simulink model "PILEncoder"  (R2021a)
settings: Solver=FixedStepAuto  StartTime=0.0  StopTime=41.24  FixedStep=0.001  RelTol=1e-3  EnableMultiTasking=on
values from neighbouring files (symbols this model uses):
  den_lpf_d = den_lpf20    [Mainframe_init.m]    (also in load_autopilot.m)
  Emulated_FCC_IO_Delay = 7    [Mainframe_init.m]
  Enable_Gyros = 0    [Mainframe_init.m]
  Enable_INS = 0    [Mainframe_init.m]
  num_lpf_d = num_lpf20    [Mainframe_init.m]    (also in load_autopilot.m)
undefined symbols (not defined in the file or in its folder): act_dmp, act_omega, Actuator, Aerodynamics, aMode, Autopilot, AUX, c_b_WGS, c_be, c_flat, c_grav, c_h_geop0, c_h_geope, c_pa0, c_pe, c_r0, c_rot, c_rsma, c_Tmp0, d_siB_0, d_siB_max, d_siB_min, dd_siB_max, dd_siB_min, dev, DiscIntNeverNeededParam, e_pa, e_Tmp, Earth, fin_maxrate, flag_I_act_switch, flag_I_aero_switch, flag_I_flat, flag_I_gravity_switch, flag_I_rot, Flight_Logic, hcr, HIL_Data, JMMM_0, JMMM_e, JSPB_e, lat_0, lon_0, Main, Mass_Props, mB_0, mM_0, mM_e, pBII_0, pMPB, pNPB, propellant_kg, prp_FBPB, prp_mdot, prp_T, pSPB, pwm_output0, pwm_output1, qEG_0, qIB_0 ... (+30)
libraries: simulink x42, simulink_extras x24, aerolibcommonsys x4, px4lib x2, custom_blocks x1, dspstat3 x1, pil_lib x1, aerolibtransform2 x1, dspnetwork x1, aerolibnav x1
(part 6 of 16)

== system PILEncoder/Non-linear Flight Dynamic Model/Subsystem1/GRM_Airframe/gravity/launch_rail ==
  gBG_c : Inport
  hBE : Inport  Port=2
  Constant1 : Constant  Value=flag_I_gravity_switch
  Constant3 : Constant  Value=0
  Subtract : Sum  Inputs=++-
  Switch : Switch  Criteria=u2 > Threshold  Threshold=0.05
  Vector Concatenate : Concatenate  NumInputs=3
  initial_altitude : Subsystem
  gBG : Outport  VectorParamsAs1DForOutWhenUnconnected=off
  wires:
  Constant1/1 -> Subtract/2
  hBE/1 -> Subtract/1
  Subtract/1 -> Switch/2
  Constant3/1 -> Vector Concatenate/1, Vector Concatenate/2, Vector Concatenate/3
  Switch/1 -> gBG/1  "gBG"
  Vector Concatenate/1 -> Switch/3
  gBG_c/1 -> Switch/1
  initial_altitude/1(hBE_0) -> Subtract/3

== system PILEncoder/Non-linear Flight Dynamic Model/Subsystem1/GRM_Airframe/motion_kinematics/calc_motion_kinematics ==
  lat : Inport
  lon : Inport  Port=2
  qIB : Inport  Port=3
  calc_transformation_matrix : Subsystem
  earth_rotation : Subsystem
  wIEE : Outport  VectorParamsAs1DForOutWhenUnconnected=off
  TIE : Outport  Port=2  VectorParamsAs1DForOutWhenUnconnected=off
  TEB : Outport  Port=3  VectorParamsAs1DForOutWhenUnconnected=off
  TGB : Outport  Port=4  VectorParamsAs1DForOutWhenUnconnected=off
  TEG : Outport  Port=5  VectorParamsAs1DForOutWhenUnconnected=off
  wEGG : Outport  Port=6  VectorParamsAs1DForOutWhenUnconnected=off
  TIB : Outport  Port=7  VectorParamsAs1DForOutWhenUnconnected=off
  wires:
  earth_rotation/1(wIEE) -> wIEE/1
  earth_rotation/2(TIE) -> TIE/1
  earth_rotation/5(TEG) -> TEG/1
  earth_rotation/6(wEGG) -> wEGG/1
  lon/1 -> earth_rotation/2(lon)
  lat/1 -> earth_rotation/1(lat)
  earth_rotation/3(qIE) -> calc_transformation_matrix/1(qIE)
  earth_rotation/4(qEG) -> calc_transformation_matrix/2(qEG)
  qIB/1 -> calc_transformation_matrix/3(qIB)
  calc_transformation_matrix/1(TEB) -> TEB/1
  calc_transformation_matrix/2(TGB) -> TGB/1
  calc_transformation_matrix/3(TIB) -> TIB/1

== system PILEncoder/Non-linear Flight Dynamic Model/Subsystem1/GRM_Airframe/propulsion/prp_look_up ==
  env_glbl_bus : Inport
  Bus Selector1 : BusSelector  OutputSignals=T_sim_glbl,T_sim_lnch
  Constant : Constant  Value=0
  Constant1 : Constant  Value=0
  Saturation : Saturate  UpperLimit=prp_T(end)  LowerLimit=0
      settings: AttributesFormatString=|
      | %<UpperLimit>
      | %<LowerLimit>
  Subtract : Sum  Inputs=+-
  Switch : Switch  Criteria=u2 > Threshold
  Switch1 : Switch  Criteria=u2 > Threshold
  Vector Concatenate : Concatenate  NumInputs=3
  thrust_lookup : Lookup_n-D  NumberOfTableDimensions=1  BreakpointsForDimension1=prp_T  Table=prp_FBPB  ExtrapMethod=Clip  UseLastTableValue=on  InternalRulePriority=Speed  RndMeth=Simplest  InputSameDT=on
  FBPM : Outport  VectorParamsAs1DForOutWhenUnconnected=off
  wires:
  Bus Selector1/2 -> Subtract/2  "<T_sim_lnch>"
  Switch/1 -> Saturation/1, Switch1/2, Switch1/3
  thrust_lookup/1 -> Switch1/1
  Bus Selector1/1 -> Subtract/1  "<T_sim_glbl>"
  env_glbl_bus/1 -> Bus Selector1/1
  Constant/1 -> Switch/3
  Subtract/1 -> Switch/1, Switch/2
  Saturation/1 -> thrust_lookup/1
  Vector Concatenate/1 -> FBPM/1  "FBPM"
  Constant1/1 -> Vector Concatenate/3, Vector Concatenate/2
  Switch1/1 -> Vector Concatenate/1  "a_FBPM"

== system PILEncoder/Non-linear Flight Dynamic Model/Subsystem1/GRM_Airframe/propulsion/prp_uncertainty ==
  FBPM : Inport
  wab : Inport  Port=2
  3_rot_mat : Subsystem  mask(Rotation um 1, 2 oder 3 Achsen){rot_1=Rotation um z-Achse, rot_2=Rotation um y-Achse, rot_3=Rotation um x-Achse}
      mask prompts: rot_1 "1. Rotation"; rot_2 "2. Rotation"; rot_3 "3. Rotation"
      mask help:
      | Dieser Block liefert die Rotationsmatrix T12 für den Fall zurück, dass sich das Ziel-Koordinatensystem (1) durch Drehungen um 1, 2 oder 3 Achsen gegenüber dem Ausgangskoordinatensystem (2) beschreiben lässt (passive Drehung).
      |
      | Die Anzahl der Rotation sowie die Reihenfolge ist frei einstellbar.
      |
      | Die Rotationswinkel haben die Einheit [rad].
      mask TypeOptions rot_1: Rotation um x-Achse | Rotation um y-Achse | Rotation um z-Achse
      mask TypeOptions rot_2: Rotation um x-Achse | Rotation um y-Achse | Rotation um z-Achse
      mask TypeOptions rot_3: Rotation um x-Achse | Rotation um y-Achse | Rotation um z-Achse
  Bus Selector : BusSelector  OutputSignals=pBPB
  Product : Product  Multiplication=Matrix(*)
  Product1 : Product
  Subtract : Sum  Inputs=+-
  Thrust_rot_z : Constant  Value=unc_prp_z
  cross_product : Subsystem
      mask help: cross product r3 = r1 x r2
      mask Help:
      | Name:
      | 
      |     cross_product
      | 
      | Description:
      | 
      |     This block implements the cross product r3 = r1 x r2.
      | 
      | Inputs  [size] [data type] [unit]:
      | 
      |     vector 1  [3] [double] [-]
      |     vector 2  [3] [double] [-]
      | 
      | Outputs  [size] [data type] [unit]:
      | 
      |     resulting vector  [3] [double] [-]
      mask Display: disp(' r3 = r1 x r2')
  pNPB : Constant  Value=pNPB
  thrust_rot_x : Constant  Value=unc_prp_x
  thrust_rot_y : Constant  Value=unc_prp_y
  uncert_thrust : Constant  Value=unc_prp_scale
  FBPB : Outport  VectorParamsAs1DForOutWhenUnconnected=off
  MBPB : Outport  Port=2  VectorParamsAs1DForOutWhenUnconnected=off
  wires:
  Thrust_rot_z/1 -> 3_rot_mat/1(wi1)
  thrust_rot_x/1 -> 3_rot_mat/3(wi3)
  Product/1 -> cross_product/2(r2), FBPB/1  "FBPB"
  FBPM/1 -> Product1/1
  3_rot_mat/1(T12) -> Product/1
  thrust_rot_y/1 -> 3_rot_mat/2(wi2)
  cross_product/1(r1_x_r2) -> MBPB/1  "MBPB"
  wab/1 -> Bus Selector/1
  Bus Selector/1 -> Subtract/1  "<pBPB>"
  uncert_thrust/1 -> Product1/2
  Product1/1 -> Product/2
  pNPB/1 -> Subtract/2
  Subtract/1 -> cross_product/1(r1)

== system PILEncoder/Non-linear Flight Dynamic Model/Subsystem1/GRM_Airframe/rb_eom/calc_bus_flight_dyn_bus_entries ==
  mot_kin : Inport
  eom : Inport  Port=2
  Bus Selector : BusSelector  OutputSignals=pBII,vBII,qIB,wBIB,d_wBIB,d_vBII
  Bus Selector1 : BusSelector  OutputSignals=pBII
  Bus Selector3 : BusSelector  OutputSignals=TGB,TIB,TIE
  Constant : Constant  Value=pBII_0
      settings: AttributesFormatString=%<Value>
  Gain : Gain  Gain=-1
  Math Function : Math  Operator=transpose  SignedPower=on  SaturateOnIntegerOverflow=on
  Product{,1..3} (4 alike) : Product  Multiplication=Matrix(*)
  Subsystem2 : Subsystem
  Sum : Sum  Inputs=+-
  eom D1 : InportShadow  Port=2
  q12_from_T12 : Subsystem
      mask help: Transforms a Direction Cosine Matrix into a Quaternion
      mask Help:
      | Name:
      | 
      |     q12_from_T12
      | 
      | Description:
      | 
      |     This block implements the transformation of a direction cosine matrix DCM
      |      into the corresponding quaternion.
      | 
      | Inputs  [size] [data type] [unit]:
      | 
      |     direction cosine matrix T12  [3x3] [double] [-]
      | 
      | Outputs  [size] [data type] [unit]:
      | 
      |     quaternion q12  [4] [double] [-]
      mask Display:
      | %port_label('input', 1, 'T12')
      | %port_label('output', 1, 'q12')
      | disp('DCM \rightarrow q','texmode','on')
  quaternion_to_euler_angles : Subsystem
      mask help: transforms quaternions to Euler angles (roll, pitch, yaw)
      mask Help:
      | Name:
      | 
      |     quaternion_to_euler_angles
      | 
      | Description:
      | 
      |     This block implements the transformation of a quaternion into the
      |     corresponding Euler angles (zyx-sequence, roll, pitch, yaw).
      | 
      | Inputs  [size] [data type] [unit]:
      | 
      |     quaternion  [4] [double] [-]
      | 
      | Outputs  [size] [data type] [unit]:
      | 
      |     roll angle phi  [1] [double] [rad]
      |     pitch angle theta  [1] [double] [rad]
      |     yaw angle psi  [1] [double] [rad]
      mask Display:
      | %disp (' q --> (Phi,Theta,Psi) [rad]')
      | disp('q \rightarrow eu(\Phi;\Theta;\Psi)','texmode','on')
  quaternion_to_euler_angles1 : Subsystem
      mask help: transforms quaternions to Euler angles (roll, pitch, yaw)
      mask Help:
      | Name:
      | 
      |     quaternion_to_euler_angles
      | 
      | Description:
      | 
      |     This block implements the transformation of a quaternion into the
      |     corresponding Euler angles (zyx-sequence, roll, pitch, yaw).
      | 
      | Inputs  [size] [data type] [unit]:
      | 
      |     quaternion  [4] [double] [-]
      | 
      | Outputs  [size] [data type] [unit]:
      | 
      |     roll angle phi  [1] [double] [rad]
      |     pitch angle theta  [1] [double] [rad]
      |     yaw angle psi  [1] [double] [rad]
      mask Display:
      | %disp (' q --> (Phi,Theta,Psi) [rad]')
      | disp('q \rightarrow eu(\Phi;\Theta;\Psi)','texmode','on')
  aBIB : Outport  VectorParamsAs1DForOutWhenUnconnected=off
  lon : Outport  Port=2  VectorParamsAs1DForOutWhenUnconnected=off
  lat : Outport  Port=3  VectorParamsAs1DForOutWhenUnconnected=off
  hBE : Outport  Port=4  VectorParamsAs1DForOutWhenUnconnected=off
  vBII : Outport  Port=5  VectorParamsAs1DForOutWhenUnconnected=off
  qIB : Outport  Port=6  VectorParamsAs1DForOutWhenUnconnected=off
  wBIB : Outport  Port=7  VectorParamsAs1DForOutWhenUnconnected=off
  d_wBIB : Outport  Port=8  VectorParamsAs1DForOutWhenUnconnected=off
  d_vBII : Outport  Port=9  VectorParamsAs1DForOutWhenUnconnected=off
  pBII : Outport  Port=10  VectorParamsAs1DForOutWhenUnconnected=off
  euIB : Outport  Port=11  VectorParamsAs1DForOutWhenUnconnected=off
  vBIB : Outport  Port=12  VectorParamsAs1DForOutWhenUnconnected=off
  qGB : Outport  Port=13  VectorParamsAs1DForOutWhenUnconnected=off
  euGB : Outport  Port=14  VectorParamsAs1DForOutWhenUnconnected=off
  euBG : Outport  Port=15  VectorParamsAs1DForOutWhenUnconnected=off
  pBLG : Outport  Port=16  VectorParamsAs1DForOutWhenUnconnected=off
  wires:
  Bus Selector/1 -> pBII/1, Subsystem2/2(pBII)  "<pBII>"
  mot_kin/1 -> Bus Selector3/1
  Bus Selector3/3 -> Subsystem2/1(TIE)  "<TIE>"
  eom/1 -> Bus Selector/1
  Math Function/1 -> [TBI], Product1/1, Product/1  "TBI"
  Bus Selector3/2 -> Math Function/1  "<TIB>"
  Bus Selector/6 -> Product/2, d_vBII/1  "<d_vBII>"
  Product/1 -> aBIB/1  "aBIB"
  Subsystem2/1(lon) -> lon/1
  Subsystem2/2(lat) -> lat/1
  Subsystem2/3(hBE) -> hBE/1  "hBE"
  Bus Selector/2 -> Product1/2, vBII/1  "<vBII>"
  Bus Selector/3 -> quaternion_to_euler_angles/1(q), qIB/1  "<qIB>"
  Bus Selector/4 -> wBIB/1  "<wBIB>"
  Bus Selector/5 -> d_wBIB/1  "<d_wBIB>"
  quaternion_to_euler_angles/1(eulx) -> euIB/1  "euIB"
  Product1/1 -> vBIB/1  "vBIB"
  Bus Selector3/1 -> [TGB], q12_from_T12/1(T12)  "<TGB>"
  q12_from_T12/1(q12) -> quaternion_to_euler_angles1/1(q), qGB/1  "qGB"
  quaternion_to_euler_angles1/1(eulx) -> euGB/1, Gain/1  "euGB"
  Gain/1 -> euBG/1  "euBG"
  eom D1/1 -> Bus Selector1/1
  Bus Selector1/1 -> Sum/1  "<pBII>"
  Constant/1 -> Sum/2
  Sum/1 -> Product3/2  "pBLI"
  [TGB] -> Product2/1
  [TBI] -> Product2/2
  Product2/1 -> Product3/1  "TGI"
  Product3/1 -> pBLG/1  "pBLG"

== system PILEncoder/Non-linear Flight Dynamic Model/Subsystem1/GRM_Airframe/rb_eom/eom_6dof ==
  for_mom : Inport
  wab : Inport  Port=2
  Bus Selector1 : BusSelector  OutputSignals=mB,JBBB
  Bus Selector2 : BusSelector  OutputSignals=FBTB,MBTB
  Constant : Constant  Value=[pBII_0; vBII_0; qIB_0; wBIB_0]
  Constant9 : Constant  Value=[0 0 0; 0 0 0; 0 0 0]
  Rigid_Body_EOM_6_DOF : Subsystem  mask{flag_Kraft=FBTB}
      mask prompts: flag_Kraft "Input Kraftvektor"
      mask help:
      | 6DOF-Bewegungsgleichungen im ECI-System mit
      | zeitvariantem Massenträgheitsmoment.
      |
      | Modell Varianten:
      | - Koordinatensystem des Kraftvektor:
      |      FBTI : Inertial System I
      |      FBTB : Körperfestes System B
      mask init:
      | switch flag_Kraft
      |     case 1
      |         port_label_kraft = 'FBTI';
      |     case 2
      |         port_label_kraft = 'FBTB';
      | end
      mask TypeOptions flag_Kraft: FBTI | FBTB
      mask DialogControl Container4 Prompt: Modell Einstellungen
      mask Display:
      | port_label ('input',1,port_label_kraft )
      | port_label ('input',2,'MBTB' )
      | port_label ('input',3,'mB' )
      | port_label ('input',4,'x0' )
      | port_label ('input',5,'JBB' )
      | port_label ('input',6,'d_JBB' )
      | port_label ('output',1,'rb_eom' )
  eom : Outport  VectorParamsAs1DForOutWhenUnconnected=off
  wires:
  Bus Selector2/2 -> Rigid_Body_EOM_6_DOF/2(MBTB)  "<MBTB>"
  Bus Selector2/1 -> Rigid_Body_EOM_6_DOF/1(FBTX)  "<FBTB>"
  Rigid_Body_EOM_6_DOF/1(rb_eom) -> eom/1
  Constant9/1 -> Rigid_Body_EOM_6_DOF/6(d_JBB)
  Bus Selector1/2 -> Rigid_Body_EOM_6_DOF/5(JBB)  "<JBBB>"
  for_mom/1 -> Bus Selector2/1
  Constant/1 -> Rigid_Body_EOM_6_DOF/4(x0)
  Bus Selector1/1 -> Rigid_Body_EOM_6_DOF/3(mB)  "<mB>"
  wab/1 -> Bus Selector1/1

== system PILEncoder/Non-linear Flight Dynamic Model/Subsystem1/GRM_Airframe/stream_flow/calc_stream_flow ==
  TIB : Inport
  wIEE : Inport  Port=2
  TIE : Inport  Port=3
  VBII : Inport  Port=4
  pBII : Inport  Port=5
  wBIB : Inport  Port=6
  rho : Inport  Port=7
  sos : Inport  Port=8
  hBE : Inport  Port=9
  Bus Creator : BusCreator  Inputs=9
  Math Function : Math  Operator=transpose  SignedPower=on  SaturateOnIntegerOverflow=on
  Product : Product  Multiplication=Matrix(*)
  Subsystem1 : Subsystem
  velocity_vector_transformation : Subsystem
  str_flow : Outport  VectorParamsAs1DForOutWhenUnconnected=off
  wires:
  Subsystem1/4(MaB) -> Bus Creator/4
  Math Function/1 -> Product/1  "TBI"
  Subsystem1/2(be) -> Bus Creator/2  "beB"
  Subsystem1/8(fi) -> Bus Creator/8  "fiB"
  VBII/1 -> velocity_vector_transformation/3(vBII)
  Subsystem1/5(a_vB) -> Bus Creator/5
  Product/1 -> Subsystem1/1(vBEB)  "vBEB"
  Subsystem1/6(wBIB_star) -> Bus Creator/6
  TIE/1 -> velocity_vector_transformation/2(TIE)
  Subsystem1/3(qdynB) -> Bus Creator/3
  velocity_vector_transformation/1(vBEI) -> Product/2
  Subsystem1/7(th) -> Bus Creator/7  "inB"
  Subsystem1/1(al) -> Bus Creator/1  "alB"
  wIEE/1 -> velocity_vector_transformation/1(wIEE)
  Bus Creator/1 -> str_flow/1  "str_flow_bus"
  wBIB/1 -> Subsystem1/2(wBIB)
  hBE/1 -> Bus Creator/9
  sos/1 -> Subsystem1/4(sos)
  rho/1 -> Subsystem1/3(rho)
  TIB/1 -> Math Function/1
  pBII/1 -> velocity_vector_transformation/4(pBII)

== system PILEncoder/Non-linear Flight Dynamic Model/Subsystem1/GRM_Airframe/weight_and_balance/center_of_gravity ==
  mB : Inport
  mM : Inport  Port=2
  1-D Lookup Table : Lookup_n-D  NumberOfTableDimensions=1  BreakpointsForDimension1=Mass_Props.propellant_bkpts  Table=Mass_Props.CGx_m_tbl  ExtrapMethod=Clip  UseLastTableValue=on  InternalRulePriority=Speed  RndMeth=Simplest  InputSameDT=on
      settings: AttributesFormatString=|
      | %<Table>
      | %<BreakpointsForDimension1>
  1-D Lookup Table3 : Lookup_n-D  NumberOfTableDimensions=1  BreakpointsForDimension1=Mass_Props.propellant_bkpts  Table=Mass_Props.CGy_m_tbl  ExtrapMethod=Clip  UseLastTableValue=on  InternalRulePriority=Speed  RndMeth=Simplest  InputSameDT=on
      settings: AttributesFormatString=|
      | %<Table>
      | %<BreakpointsForDimension1>
  1-D Lookup Table6 : Lookup_n-D  NumberOfTableDimensions=1  BreakpointsForDimension1=Mass_Props.propellant_bkpts  Table=Mass_Props.CGz_m_tbl  ExtrapMethod=Clip  UseLastTableValue=on  InternalRulePriority=Speed  RndMeth=Simplest  InputSameDT=on
      settings: AttributesFormatString=|
      | %<Table>
      | %<BreakpointsForDimension1>
  Add6 : Sum
  Add7 : Sum
  Add8 : Sum
  Constant10 : Constant  Value=unc_cg_x
  Constant11 : Constant  Value=unc_cg_y
  Constant12 : Constant  Value=unc_cg_z
  Terminator1 : Terminator
  Vector Concatenate1 : Concatenate  NumInputs=3
  mM D2 : InportShadow  Port=2
  mM D3 : InportShadow  Port=2
  pBPB : Outport  VectorParamsAs1DForOutWhenUnconnected=off
  wires:
  1-D Lookup Table6/1 -> Add8/1
  1-D Lookup Table3/1 -> Add7/1
  Vector Concatenate1/1 -> pBPB/1  "pBPB"
  1-D Lookup Table/1 -> Add6/1
  mM/1 -> 1-D Lookup Table/1
  mM D2/1 -> 1-D Lookup Table3/1
  mM D3/1 -> 1-D Lookup Table6/1
  Add6/1 -> Vector Concatenate1/1
  Constant10/1 -> Add6/2
  Constant11/1 -> Add7/2
  Add7/1 -> Vector Concatenate1/2
  Constant12/1 -> Add8/2
  Add8/1 -> Vector Concatenate1/3
  mB/1 -> Terminator1/1

== system PILEncoder/Non-linear Flight Dynamic Model/Subsystem1/GRM_Airframe/weight_and_balance/mass ==
  sim_time_launch : Inport
  1-D Lookup Table2 : Lookup_n-D  NumberOfTableDimensions=1  BreakpointsForDimension1=prp_T  Table=prp_mdot  ExtrapMethod=Clip  DiagnosticForOutOfRangeInput=Warning  UseLastTableValue=on  InternalRulePriority=Speed  RndMeth=Simplest  InputSameDT=on
  Constant : Constant  Value=0
  Constant1 : Constant  Value=mB_0
  Constant2 : Constant  Value=propellant_kg
      settings: AttributesFormatString=%<Value>
  Gain : Gain  Gain=-1
  Integrator1 : Integrator  InitialConditionSource=external
  Saturation : Saturate  UpperLimit=prp_T(end)  LowerLimit=0
      settings: AttributesFormatString=|
      | %<UpperLimit>
      | %<LowerLimit>
  Subtract1 : Sum
  Switch : Switch  Criteria=u2 > Threshold
  Switch1 : Switch  Criteria=u2 > Threshold
  mB_c : Outport  VectorParamsAs1DForOutWhenUnconnected=off
  mM : Outport  Port=2  VectorParamsAs1DForOutWhenUnconnected=off
  wires:
  Constant1/1 -> Subtract1/1
  Subtract1/1 -> mB_c/1  "mB_c"
  Switch/1 -> Switch1/2, Switch1/3, Saturation/1
  Constant/1 -> Switch/3
  sim_time_launch/1 -> Switch/1, Switch/2
  Saturation/1 -> 1-D Lookup Table2/1
  Switch1/1 -> mM/1, Subtract1/2  "mM"
  Constant2/1 -> Integrator1/2
  1-D Lookup Table2/1 -> Gain/1  "mdot_kgps"
  Gain/1 -> Integrator1/1
  Integrator1/1 -> Switch1/1  "propellant_remaining_kg"

== system PILEncoder/Non-linear Flight Dynamic Model/Subsystem1/GRM_Airframe/weight_and_balance/mass_uncertainty ==
  mB_c : Inport
  Add : Sum
  Constant : Constant  Value=unc_mB_bl
  Constant1 : Constant  Value=unc_mB_scale
  Product : Product
  mB : Outport  VectorParamsAs1DForOutWhenUnconnected=off
  wires:
  Constant/1 -> Add/1
  mB_c/1 -> Product/1
  Add/1 -> mB/1  "mB"
  Constant1/1 -> Product/2
  Product/1 -> Add/2

== system PILEncoder/Non-linear Flight Dynamic Model/Subsystem1/GRM_Airframe/weight_and_balance/moi ==
  pBPB : Inport
  mM : Inport  Port=2
  1-D Lookup Table : Lookup_n-D  NumberOfTableDimensions=1  BreakpointsForDimension1=Mass_Props.propellant_bkpts  Table=Mass_Props.Ixx_tbl  ExtrapMethod=Clip  UseLastTableValue=on  InternalRulePriority=Speed  RndMeth=Simplest  InputSameDT=on
      settings: AttributesFormatString=|
      | %<Table>
      | %<BreakpointsForDimension1>
  1-D Lookup Table1 : Lookup_n-D  NumberOfTableDimensions=1  BreakpointsForDimension1=Mass_Props.propellant_bkpts  Table=Mass_Props.Ixy_tbl  ExtrapMethod=Clip  UseLastTableValue=on  InternalRulePriority=Speed  RndMeth=Simplest  InputSameDT=on
      settings: AttributesFormatString=|
      | %<Table>
      | %<BreakpointsForDimension1>
  1-D Lookup Table2 : Lookup_n-D  NumberOfTableDimensions=1  BreakpointsForDimension1=Mass_Props.propellant_bkpts  Table=Mass_Props.Ixz_tbl  ExtrapMethod=Clip  UseLastTableValue=on  InternalRulePriority=Speed  RndMeth=Simplest  InputSameDT=on
      settings: AttributesFormatString=|
      | %<Table>
      | %<BreakpointsForDimension1>
  1-D Lookup Table3 : Lookup_n-D  NumberOfTableDimensions=1  BreakpointsForDimension1=Mass_Props.propellant_bkpts  Table=Mass_Props.Iyx_tbl  ExtrapMethod=Clip  UseLastTableValue=on  InternalRulePriority=Speed  RndMeth=Simplest  InputSameDT=on
      settings: AttributesFormatString=|
      | %<Table>
      | %<BreakpointsForDimension1>
  1-D Lookup Table4 : Lookup_n-D  NumberOfTableDimensions=1  BreakpointsForDimension1=Mass_Props.propellant_bkpts  Table=Mass_Props.Iyy_tbl  ExtrapMethod=Clip  UseLastTableValue=on  InternalRulePriority=Speed  RndMeth=Simplest  InputSameDT=on
      settings: AttributesFormatString=|
      | %<Table>
      | %<BreakpointsForDimension1>
  1-D Lookup Table5 : Lookup_n-D  NumberOfTableDimensions=1  BreakpointsForDimension1=Mass_Props.propellant_bkpts  Table=Mass_Props.Iyz_tbl  ExtrapMethod=Clip  UseLastTableValue=on  InternalRulePriority=Speed  RndMeth=Simplest  InputSameDT=on
      settings: AttributesFormatString=|
      | %<Table>
      | %<BreakpointsForDimension1>
  1-D Lookup Table6 : Lookup_n-D  NumberOfTableDimensions=1  BreakpointsForDimension1=Mass_Props.propellant_bkpts  Table=Mass_Props.Izx_tbl  ExtrapMethod=Clip  UseLastTableValue=on  InternalRulePriority=Speed  RndMeth=Simplest  InputSameDT=on
      settings: AttributesFormatString=|
      | %<Table>
      | %<BreakpointsForDimension1>
  1-D Lookup Table7 : Lookup_n-D  NumberOfTableDimensions=1  BreakpointsForDimension1=Mass_Props.propellant_bkpts  Table=Mass_Props.Izy_tbl  ExtrapMethod=Clip  UseLastTableValue=on  InternalRulePriority=Speed  RndMeth=Simplest  InputSameDT=on
      settings: AttributesFormatString=|
      | %<Table>
      | %<BreakpointsForDimension1>
  1-D Lookup Table8 : Lookup_n-D  NumberOfTableDimensions=1  BreakpointsForDimension1=Mass_Props.propellant_bkpts  Table=Mass_Props.Izz_tbl  ExtrapMethod=Clip  UseLastTableValue=on  InternalRulePriority=Speed  RndMeth=Simplest  InputSameDT=on
      settings: AttributesFormatString=|
      | %<Table>
      | %<BreakpointsForDimension1>
  Add : Sum  Commented=on
  Add4 : Sum  Commented=on
  Add5 : Sum  Commented=on
  Constant15 : Constant  Commented=on  Value=JSPB_e
  JMMM_linear_interpolation : Subsystem  Commented=on
  Matrix Concatenate : Concatenate  NumInputs=3  Mode=Multidimensional array  ConcatenateDimension=2
  Terminator : Terminator  Commented=on
  Vector Concatenate : Concatenate  NumInputs=3
  Vector Concatenate1 : Concatenate  NumInputs=3
  Vector Concatenate2 : Concatenate  NumInputs=3
  mM D{1..9} (9 alike) : InportShadow  Port=2
  moi_coordinate_transformation : Subsystem  Commented=on
  moi_uncertainty : Subsystem
  steiners_theorem_missile : Subsystem  Commented=on
  steiners_theorem_motor : Subsystem  Commented=on
  JBBB : Outport  VectorParamsAs1DForOutWhenUnconnected=off
  wires:
  mM/1 -> steiners_theorem_motor/2(mM), JMMM_linear_interpolation/1(mM)
  JMMM_linear_interpolation/1(JMMM) -> moi_coordinate_transformation/1(JMMM)
  moi_coordinate_transformation/1(JMMB) -> Add/2
  pBPB/1 -> steiners_theorem_missile/1(pBPB), steiners_theorem_motor/1(pBPB)
  steiners_theorem_motor/1(JM_deviation) -> Add/1
  Add/1 -> Add4/2  "JMBB"
  Constant15/1 -> Add5/1
  Add5/1 -> Add4/1  "JSBB"
  steiners_theorem_missile/1(J_deviation) -> Add5/2
  Add4/1 -> Terminator/1  "JBBB_c"
  moi_uncertainty/1(JBBB) -> JBBB/1
  mM D1/1 -> 1-D Lookup Table/1
  mM D2/1 -> 1-D Lookup Table3/1
  mM D3/1 -> 1-D Lookup Table6/1
  mM D4/1 -> 1-D Lookup Table1/1
  mM D5/1 -> 1-D Lookup Table4/1
  mM D6/1 -> 1-D Lookup Table7/1
  mM D7/1 -> 1-D Lookup Table2/1
  mM D8/1 -> 1-D Lookup Table5/1
  mM D9/1 -> 1-D Lookup Table8/1
  1-D Lookup Table6/1 -> Vector Concatenate/3
  1-D Lookup Table3/1 -> Vector Concatenate/2
  1-D Lookup Table/1 -> Vector Concatenate/1
  1-D Lookup Table1/1 -> Vector Concatenate1/1
  1-D Lookup Table4/1 -> Vector Concatenate1/2
  1-D Lookup Table7/1 -> Vector Concatenate1/3
  1-D Lookup Table2/1 -> Vector Concatenate2/1
  1-D Lookup Table5/1 -> Vector Concatenate2/2
  1-D Lookup Table8/1 -> Vector Concatenate2/3
  Vector Concatenate/1 -> [MOI_matrix_col1]
  Vector Concatenate1/1 -> [MOI_matrix_col2]
  Vector Concatenate2/1 -> [MOI_matrix_col3]
  [MOI_matrix_col1] -> Matrix Concatenate/1
  [MOI_matrix_col2] -> Matrix Concatenate/2
  [MOI_matrix_col3] -> Matrix Concatenate/3
  Matrix Concatenate/1 -> moi_uncertainty/1(JBBB_c)  "JBBB_c"

== system PILEncoder/Flight Control Computer/FCC - Real or Emulated/Emulated FCC/P2R5/Emulated Pixhawk/Autopilot ==
  Cmd : Inport
  IMU Data : Inport  Port=2
  INS Data : Inport  Port=3
  Trigger : TriggerPort  VariantControl=Variant  PortDimensions=1
  Bus Selector3 : BusSelector  OutputSignals=p,q,r
  Bus Selector4 : BusSelector  OutputSignals=acc_x,acc_y,acc_z
  Bus Selector5 : BusSelector  OutputSignals=phi,z,w
  Calculate U1 : Subsystem
  Constant{,1..8} (9 alike) : Constant  Value=0
  Flight_Software : Subsystem
  From4 : From  Commented=on  GotoTag=rst  TagVisibility=global
  Gain1 : Gain  Gain=-1
  Fin Deflections : Outport
  flight_mode_enum : Outport  Port=2
  Fin Cmd : Outport  Port=3  VectorParamsAs1DForOutWhenUnconnected=off
  Recovery : Outport  Port=4
  wires:
  IMU Data/1 -> Bus Selector4/1
  INS Data/1 -> Bus Selector3/1, Calculate U1/1(INS Data), Bus Selector5/1
  Bus Selector4/1 -> Flight_Software/1(IMU_Ax_mps2)  "<acc_x>"
  Bus Selector4/2 -> Flight_Software/2(IMU_Ay_mps2)  "<acc_y>"
  Bus Selector4/3 -> Flight_Software/3(IMU_Az_mps2)  "<acc_z>"
  Bus Selector5/1 -> Flight_Software/7(phi_fb_rad)  "<phi>"
  Calculate U1/1(U) -> Flight_Software/8(V_mps)
  Bus Selector3/1 -> Flight_Software/4(IMU_p_rps)  "<p>"
  Bus Selector3/2 -> Flight_Software/5(IMU_q_rps)  "<q>"
  Bus Selector3/3 -> Flight_Software/6(IMU_r_rps)  "<r>"
  Bus Selector5/2 -> Gain1/1  "<z>"
  Bus Selector5/3 -> Flight_Software/10(Vz_mps)  "<w>"
  Constant5/1 -> Flight_Software/18(gcs_RTL_log)
  Constant4/1 -> Flight_Software/17(gcs_traj_cmd_enum)
  Constant3/1 -> Flight_Software/16(gcs_integrators_on)
  Constant2/1 -> Flight_Software/15(gcs_fin4_cmd_deg)
  Constant1/1 -> Flight_Software/14(gcs_fin3_cmd_deg)
  Constant/1 -> Flight_Software/13(gcs_fin2_cmd_deg)
  Constant6/1 -> Flight_Software/11(gcs_manual_fin_cmds_log)
  Constant7/1 -> Flight_Software/12(gcs_fin1_cmd_deg)
  Gain1/1 -> Flight_Software/9(h_m)
  Cmd/1 -> Flight_Software/20(Phi_cmd)
  Flight_Software/1(Fin Cmd) -> Fin Deflections/1, Fin Cmd/1
  Flight_Software/2(flight_mode_enum) -> flight_mode_enum/1
  Flight_Software/3(Recovery) -> Recovery/1
  Constant8/1 -> Flight_Software/19(Reset Integrators)

== system PILEncoder/Flight Control Computer/FCC - Real or Emulated/Emulated FCC/P2R5/Emulated Pixhawk/Convert to Bus ==
  Input : Inport  OutDataTypeStr=single
  100Hz Reset : Subsystem
  Bus Creator1 : BusCreator  Inputs=6
  Bus Creator2 : BusCreator  Inputs=12
  Bus Creator3 : BusCreator  Inputs=1
  Demux : Demux  Outputs=23
  Heartbeat : Outport  InitialOutput=0
  Ext. Commands : Outport  Port=2  OutDataTypeStr=single  InitialOutput=0
  Enable INS Flag : Outport  Port=3  InitialOutput=0
  Missile States : Outport  Port=4  OutDataTypeStr=single  InitialOutput=[0 0 0 0 0 0 0 0 0 0]
  Real Gyros Flag : Outport  Port=5  InitialOutput=0
  Virtual IMU Data : Outport  Port=6  OutDataTypeStr=single  InitialOutput=[0 0 0 0 0 0 0 0 0 0]
  tag scope: FCC_Enable=global, rst=global
  wires:
  Demux/22 -> Bus Creator2/12  "psi"
  Demux/21 -> Bus Creator2/11  "theta"
  Demux/20 -> Bus Creator2/10  "phi"
  Demux/4 -> Real Gyros Flag/1  "Real Gyros Flag"
  Demux/5 -> Bus Creator2/1  "u"
  Demux/18 -> Bus Creator1/5  "gyro_y"
  Bus Creator1/1 -> Virtual IMU Data/1
  Demux/16 -> Bus Creator1/3  "acc_z"
  Demux/9 -> Bus Creator2/5  "y"
  Demux/14 -> Bus Creator1/1  "acc_x"
  Demux/17 -> Bus Creator1/4  "gyro_x"
  Demux/15 -> Bus Creator1/2  "acc_y"
  Demux/19 -> Bus Creator1/6  "gyro_z"
  Demux/12 -> Bus Creator2/8  "q"
  Demux/7 -> Bus Creator2/3  "w"
  Demux/10 -> Bus Creator2/6  "z"
  Demux/6 -> Bus Creator2/2  "v"
  Demux/11 -> Bus Creator2/7  "p"
  Demux/13 -> Bus Creator2/9  "r"
  Demux/23 -> Bus Creator3/1  "phi_cmd"
  Demux/8 -> Bus Creator2/4  "x"
  Bus Creator3/1 -> Ext. Commands/1
  Bus Creator2/1 -> Missile States/1
  Demux/1 -> [FCC_Enable]  "EnableFCC"
  Input/1 -> Demux/1
  Demux/2 -> 100Hz Reset/1(Heartbeat), Heartbeat/1  "Hearbeat"
  Demux/3 -> Enable INS Flag/1  "Enable INS Flag"
  100Hz Reset/1(RST) -> [rst]

== system PILEncoder/Flight Control Computer/FCC - Real or Emulated/Emulated FCC/P2R5/Emulated Pixhawk/Convert to Vector ==
  Fin Deflections : Inport
  Heartbeat : Inport  Port=2
  INS Data : Inport  Port=3
  Real Gyro Data : Inport  Port=4
  Debug Port : Inport  Port=5
  Bus Selector1 : BusSelector  OutputSignals=Fin_1_Cmd_rad,Fin_2_Cmd_rad,Fin_3_Cmd_rad,Fin_4_Cmd_rad
  Bus Selector2 : BusSelector  OutputSignals=gyro_x,gyro_y,gyro_z
  Bus Selector3 : BusSelector  OutputSignals=u,v,w,x,y,z,p,q,r
  Cast To Single : DataTypeConversion  OutDataTypeStr=single
  Vector Concatenate : Concatenate  NumInputs=18
  To HIL : Outport
  wires:
  Bus Selector1/3 -> Vector Concatenate/4  "<Fin_3_Cmd_rad>"
  Bus Selector1/4 -> Vector Concatenate/5  "<Fin_4_Cmd_rad>"
  Heartbeat/1 -> Vector Concatenate/1
  Bus Selector1/1 -> Vector Concatenate/2  "<Fin_1_Cmd_rad>"
  Bus Selector1/2 -> Vector Concatenate/3  "<Fin_2_Cmd_rad>"
  Vector Concatenate/1 -> Cast To Single/1
  Fin Deflections/1 -> Bus Selector1/1
  Cast To Single/1 -> To HIL/1
  Real Gyro Data/1 -> Bus Selector2/1
  Bus Selector3/7 -> Vector Concatenate/15  "<p>"
  Bus Selector3/5 -> Vector Concatenate/13  "<y>"
  Bus Selector3/4 -> Vector Concatenate/12  "<x>"
  Bus Selector3/9 -> Vector Concatenate/17  "<r>"
  Bus Selector3/3 -> Vector Concatenate/11  "<w>"
  Bus Selector2/3 -> Vector Concatenate/8  "<gyro_z>"
  Debug Port/1 -> Vector Concatenate/18
  Bus Selector3/1 -> Vector Concatenate/9  "<u>"
  Bus Selector2/2 -> Vector Concatenate/7  "<gyro_y>"
  Bus Selector2/1 -> Vector Concatenate/6  "<gyro_x>"
  Bus Selector3/8 -> Vector Concatenate/16  "<q>"
  INS Data/1 -> Bus Selector3/1
  Bus Selector3/6 -> Vector Concatenate/14  "<z>"
  Bus Selector3/2 -> Vector Concatenate/10  "<v>"

== system PILEncoder/Flight Control Computer/FCC - Real or Emulated/Emulated FCC/P2R5/Emulated Pixhawk/IMU - Merge ==
  HIL IMU : Inport
  Bus Creator2 : BusCreator  Inputs=6
  Bus Selector2 : BusSelector  OutputSignals=acc_x,acc_y,acc_z,gyro_x,gyro_y,gyro_z
  IMU Data : Outport
  wires:
  HIL IMU/1 -> Bus Selector2/1
  Bus Selector2/5 -> Bus Creator2/5  "<gyro_y>"
  Bus Selector2/6 -> Bus Creator2/6  "<gyro_z>"
  Bus Selector2/4 -> Bus Creator2/4  "<gyro_x>"
  Bus Selector2/2 -> Bus Creator2/2  "<acc_y>"
  Bus Selector2/1 -> Bus Creator2/1  "<acc_x>"
  Bus Selector2/3 -> Bus Creator2/3  "<acc_z>"
  Bus Creator2/1 -> IMU Data/1

== system PILEncoder/Flight Control Computer/FCC - Real or Emulated/Emulated FCC/P2R5/Emulated Pixhawk/Inertial Navigation System ==
  Enable INS Flag : Inport
  Missile States : Inport  Port=2
  IMU Data : Inport  Port=3
  INS (INCOMPLETE) : Subsystem
  Switch : Switch  Criteria=u2 > Threshold
  INS Data : Outport
  wires:
  Enable INS Flag/1 -> Switch/2
  IMU Data/1 -> INS (INCOMPLETE)/1(IMU Data)
  Switch/1 -> INS Data/1
  Missile States/1 -> Switch/3
  INS (INCOMPLETE)/1(INS Data) -> Switch/1

== system PILEncoder/Flight Control Computer/FCC - Real or Emulated/Emulated FCC/P2R5/Emulated Pixhawk/Real Gyro ==
  HIL Gyro : Inport
  Bus Creator2 : BusCreator  Inputs=3
  Bus Selector2 : BusSelector  OutputSignals=gyro_x,gyro_y,gyro_z
  Gyro Data : Outport
  wires:
  HIL Gyro/1 -> Bus Selector2/1
  Bus Selector2/2 -> Bus Creator2/2  "<gyro_y>"
  Bus Selector2/1 -> Bus Creator2/1  "<gyro_x>"
  Bus Selector2/3 -> Bus Creator2/3  "<gyro_z>"
  Bus Creator2/1 -> Gyro Data/1

== system PILEncoder/Flight Control Computer/FCC - Real or Emulated/Emulated FCC/P2R5/Emulated Pixhawk/Servo Commands ==
  Fin Cmd : Inport
  Recovery : Inport  Port=2
  100Hz Progress : Subsystem
  AND : Logic  IconShape=distinctive  AllPortsSameDT=off  OutDataTypeStr=boolean
  Add{,1..3} (4 alike) : Sum
  Bus Selector : BusSelector  OutputSignals=Fin_1_Cmd_rad,Fin_2_Cmd_rad,Fin_3_Cmd_rad,Fin_4_Cmd_rad
  Cast To Boolean : DataTypeConversion  OutDataTypeStr=boolean
  Cast To Double{,1..4} (5 alike) : DataTypeConversion  OutDataTypeStr=uint16
  Gain{,1..3} (4 alike) : Gain  Gain=1000/91
  One{,1..3} (4 alike) : Constant  Value=900  OutDataTypeStr=Inherit: Inherit via back propagation
  One4 : Constant  Value=0  OutDataTypeStr=boolean
  One5 : Constant  Value=2000  OutDataTypeStr=Inherit: Inherit via back propagation
  One6 : Constant  Value=1000  OutDataTypeStr=Inherit: Inherit via back propagation
  One7 : Constant  OutDataTypeStr=boolean
  PX4 PWM Output1 : px4lib/PX4 PWM Output  pwmDevice=Main (/dev/pwm_output0)  pwmChannel1_=on  pwmChannel2_=on  pwmChannel3_=on  pwmChannel4_=on  pwmChannel5_=on  pwmChannel6_=off  pwmChannel7_=off  pwmChannel8_=off  forceTerminateFailsafe=off  outputErrorStatus=off
      settings: SourceProductBaseCode=PX4AUTOPILOTS
  Radians to Degrees{,1..3} (4 alike) : simulink_extras/Transformations/Radians to Degrees
  Saturation{,1..3} (4 alike) : Saturate  UpperLimit=20  LowerLimit=-20
  Switch : Switch  Criteria=u2 > Threshold
  Terminator : Terminator
  wires:
  Saturation2/1 -> Gain2/1
  Cast To Double3/1 -> PX4 PWM Output1/6
  One4/1 -> PX4 PWM Output1/2
  One/1 -> Add/2
  One2/1 -> Add2/2
  Add1/1 -> Cast To Double1/1
  Gain2/1 -> Add2/1
  AND/1 -> Cast To Boolean/1
  Radians to Degrees1/1 -> Saturation1/1
  Cast To Double2/1 -> PX4 PWM Output1/5
  Add2/1 -> Cast To Double2/1
  Fin Cmd/1 -> Bus Selector/1
  Cast To Double1/1 -> PX4 PWM Output1/4
  Bus Selector/2 -> Radians to Degrees1/1  "<Fin_2_Cmd_rad>"
  Gain/1 -> Add/1
  Bus Selector/4 -> Radians to Degrees3/1  "<Fin_4_Cmd_rad>"
  One3/1 -> Add3/2
  Saturation/1 -> Gain/1
  Gain1/1 -> Add1/1
  Saturation3/1 -> Gain3/1
  Gain3/1 -> Add3/1
  Radians to Degrees3/1 -> Saturation3/1
  Bus Selector/1 -> Radians to Degrees/1  "<Fin_1_Cmd_rad>"
  Bus Selector/3 -> Radians to Degrees2/1  "<Fin_3_Cmd_rad>"
  Saturation1/1 -> Gain1/1
  Cast To Double/1 -> PX4 PWM Output1/3
  Add3/1 -> Cast To Double3/1
  Radians to Degrees2/1 -> Saturation2/1
  [FCC_Enable] -> AND/1
  Radians to Degrees/1 -> Saturation/1
  100Hz Progress/1(RST) -> AND/2
  One1/1 -> Add1/2
  Add/1 -> Cast To Double/1
  Cast To Double4/1 -> PX4 PWM Output1/7
  Recovery/1 -> Switch/2
  One5/1 -> Switch/1
  One6/1 -> Switch/3
  Switch/1 -> Cast To Double4/1
  Cast To Boolean/1 -> Terminator/1
  One7/1 -> PX4 PWM Output1/1

== system PILEncoder/Flight Control Computer/FCC - Real or Emulated/Real FCC/PixBlock2/Emulated Pixhawk/Autopilot ==
  Cmd : Inport
  IMU Data : Inport  Port=2
  INS Data : Inport  Port=3
  Bus Creator3 : BusCreator  Inputs=3
  Bus Selector : BusSelector  OutputSignals=phi_cmd
  Bus Selector1 : BusSelector  OutputSignals=gyro_x
  Bus Selector2 : BusSelector  OutputSignals=phi,z,p
  Calculate U : Subsystem
  Discrete Transfer Fcn : DiscreteTransferFcn  Numerator=[num_lpf_d]  Denominator=[den_lpf_d]
  Gain : Gain  Gain=-1
  Manual Switch : ManualSwitch
  Phi_Control : Subsystem
  Zero : Constant  Value=0  OutDataTypeStr=Inherit: Inherit via back propagation
  Attitude_Commands : Outport  VectorParamsAs1DForOutWhenUnconnected=off
  wires:
  Bus Selector1/1 -> Discrete Transfer Fcn/1  "<gyro_x>"
  IMU Data/1 -> Bus Selector1/1
  Calculate U/1(U) -> Phi_Control/5(V_mps)
  Zero/1 -> [Delta_Cmd_Psi], [Delta_Cmd_Theta]
  [Delta_Cmd_Phi] -> Bus Creator3/1  "Phi_Cmd_rad"
  [Delta_Cmd_Theta] -> Bus Creator3/2  "Theta_Cmd_rad"
  Bus Creator3/1 -> Attitude_Commands/1
  [Delta_Cmd_Psi] -> Bus Creator3/3  "Psi_Cmd_rad"
  Bus Selector/1 -> Phi_Control/1(phi_cmd_rad)  "<phi_cmd>"
  Cmd/1 -> Bus Selector/1
  INS Data/1 -> Calculate U/1(INS Data), Bus Selector2/1
  Bus Selector2/1 -> Phi_Control/2(phi_rad)  "<phi>"
  [rst] -> Phi_Control/4(Reset Integrators)
  Bus Selector2/2 -> Gain/1  "<z>"
  Gain/1 -> Phi_Control/6(h_m)
  Phi_Control/1(dela_cmd_rad) -> [Delta_Cmd_Phi]  "Phi_Cmd_rad"
  Discrete Transfer Fcn/1 -> Manual Switch/1
  Bus Selector2/3 -> Manual Switch/2  "<p>"
  Manual Switch/1 -> Phi_Control/3(p_rps)

== system PILEncoder/Flight Control Computer/FCC - Real or Emulated/Real FCC/PixBlock2/Emulated Pixhawk/Convert to Bus ==
  Input : Inport  OutDataTypeStr=single
  100Hz Reset : Subsystem
  Bus Creator1 : BusCreator  Inputs=6
  Bus Creator2 : BusCreator  Inputs=12
  Bus Creator3 : BusCreator  Inputs=1
  Demux : Demux  Outputs=23
  Heartbeat : Outport  InitialOutput=0
  Ext. Commands : Outport  Port=2  OutDataTypeStr=single  InitialOutput=0
  Enable INS Flag : Outport  Port=3  InitialOutput=0
  Missile States : Outport  Port=4  OutDataTypeStr=single  InitialOutput=[0 0 0 0 0 0 0 0 0 0]
  Real Gyros Flag : Outport  Port=5  InitialOutput=0
  Virtual IMU Data : Outport  Port=6  OutDataTypeStr=single  InitialOutput=[0 0 0 0 0 0 0 0 0 0]
  tag scope: FCC_Enable=global, rst=global
  wires:
  Demux/22 -> Bus Creator2/12  "psi"
  Demux/21 -> Bus Creator2/11  "theta"
  Demux/20 -> Bus Creator2/10  "phi"
  Demux/4 -> Real Gyros Flag/1  "Real Gyros Flag"
  Demux/5 -> Bus Creator2/1  "u"
  Demux/18 -> Bus Creator1/5  "gyro_y"
  Bus Creator1/1 -> Virtual IMU Data/1
  Demux/16 -> Bus Creator1/3  "acc_z"
  Demux/9 -> Bus Creator2/5  "y"
  Demux/14 -> Bus Creator1/1  "acc_x"
  Demux/17 -> Bus Creator1/4  "gyro_x"
  Demux/15 -> Bus Creator1/2  "acc_y"
  Demux/19 -> Bus Creator1/6  "gyro_z"
  Demux/12 -> Bus Creator2/8  "q"
  Demux/7 -> Bus Creator2/3  "w"
  Demux/10 -> Bus Creator2/6  "z"
  Demux/6 -> Bus Creator2/2  "v"
  Demux/11 -> Bus Creator2/7  "p"
  Demux/13 -> Bus Creator2/9  "r"
  Demux/23 -> Bus Creator3/1  "phi_cmd"
  Demux/8 -> Bus Creator2/4  "x"
  Bus Creator3/1 -> Ext. Commands/1
  Bus Creator2/1 -> Missile States/1
  Demux/1 -> [FCC_Enable]  "EnableFCC"
  Input/1 -> Demux/1
  Demux/2 -> 100Hz Reset/1(Heartbeat), Heartbeat/1  "Hearbeat"
  Demux/3 -> Enable INS Flag/1  "Enable INS Flag"
  100Hz Reset/1(RST) -> [rst]

== system PILEncoder/Flight Control Computer/FCC - Real or Emulated/Real FCC/PixBlock2/Emulated Pixhawk/Convert to Vector ==
  Fin Deflections : Inport
  Heartbeat : Inport  Port=2
  INS Data : Inport  Port=3
  Real Gyro Data : Inport  Port=4
  Debug Port : Inport  Port=5
  Bus Selector1 : BusSelector  OutputSignals=Fin_1_Cmd_rad,Fin_2_Cmd_rad,Fin_3_Cmd_rad,Fin_4_Cmd_rad
  Bus Selector2 : BusSelector  OutputSignals=gyro_x,gyro_y,gyro_z
  Bus Selector3 : BusSelector  OutputSignals=u,v,w,x,y,z,p,q,r
  Cast To Single : DataTypeConversion  OutDataTypeStr=single
  Vector Concatenate : Concatenate  NumInputs=18
  To HIL : Outport
  wires:
  Bus Selector1/3 -> Vector Concatenate/4  "<Fin_3_Cmd_rad>"
  Bus Selector1/4 -> Vector Concatenate/5  "<Fin_4_Cmd_rad>"
  Heartbeat/1 -> Vector Concatenate/1
  Bus Selector1/1 -> Vector Concatenate/2  "<Fin_1_Cmd_rad>"
  Bus Selector1/2 -> Vector Concatenate/3  "<Fin_2_Cmd_rad>"
  Vector Concatenate/1 -> Cast To Single/1
  Fin Deflections/1 -> Bus Selector1/1
  Cast To Single/1 -> To HIL/1
  Real Gyro Data/1 -> Bus Selector2/1
  Bus Selector3/7 -> Vector Concatenate/15  "<p>"
  Bus Selector3/5 -> Vector Concatenate/13  "<y>"
  Bus Selector3/4 -> Vector Concatenate/12  "<x>"
  Bus Selector3/9 -> Vector Concatenate/17  "<r>"
  Bus Selector3/3 -> Vector Concatenate/11  "<w>"
  Bus Selector2/3 -> Vector Concatenate/8  "<gyro_z>"
  Debug Port/1 -> Vector Concatenate/18
  Bus Selector3/1 -> Vector Concatenate/9  "<u>"
  Bus Selector2/2 -> Vector Concatenate/7  "<gyro_y>"
  Bus Selector2/1 -> Vector Concatenate/6  "<gyro_x>"
  Bus Selector3/8 -> Vector Concatenate/16  "<q>"
  INS Data/1 -> Bus Selector3/1
  Bus Selector3/6 -> Vector Concatenate/14  "<z>"
  Bus Selector3/2 -> Vector Concatenate/10  "<v>"

== system PILEncoder/Flight Control Computer/FCC - Real or Emulated/Real FCC/PixBlock2/Emulated Pixhawk/Fin Allocation ==
  Attitude Cmd : Inport
  Bus Creator : BusCreator  Inputs=4
  Bus Selector : BusSelector  OutputSignals=Phi_Cmd_rad,Theta_Cmd_rad,Psi_Cmd_rad
  Demux : Demux
  Vector Concatenate1 : Concatenate  NumInputs=3
  control_allocation : Subsystem
  Fin Cmd : Outport  VectorParamsAs1DForOutWhenUnconnected=off
  wires:
  Demux/4 -> Bus Creator/4  "Fin_4_Cmd_rad"
  control_allocation/1(siB_cmd) -> Demux/1
  Bus Selector/3 -> Vector Concatenate1/3  "<Psi_Cmd_rad>"
  Vector Concatenate1/1 -> control_allocation/1(fin_cmd)  "fin_cmd"
  Bus Selector/1 -> Vector Concatenate1/1  "<Phi_Cmd_rad>"
  Demux/3 -> Bus Creator/3  "Fin_3_Cmd_rad"
  Bus Selector/2 -> Vector Concatenate1/2  "<Theta_Cmd_rad>"
  Demux/1 -> Bus Creator/1  "Fin_1_Cmd_rad"
  Bus Creator/1 -> Fin Cmd/1
  Attitude Cmd/1 -> Bus Selector/1
  Demux/2 -> Bus Creator/2  "Fin_2_Cmd_rad"

== system PILEncoder/Flight Control Computer/FCC - Real or Emulated/Real FCC/PixBlock2/Emulated Pixhawk/IMU - Merge ==
  HIL IMU : Inport
  Bus Creator2 : BusCreator  Inputs=6
  Bus Selector2 : BusSelector  OutputSignals=acc_x,acc_y,acc_z,gyro_x,gyro_y,gyro_z
  IMU Data : Outport
  wires:
  HIL IMU/1 -> Bus Selector2/1
  Bus Selector2/5 -> Bus Creator2/5  "<gyro_y>"
  Bus Selector2/6 -> Bus Creator2/6  "<gyro_z>"
  Bus Selector2/4 -> Bus Creator2/4  "<gyro_x>"
  Bus Selector2/2 -> Bus Creator2/2  "<acc_y>"
  Bus Selector2/1 -> Bus Creator2/1  "<acc_x>"
  Bus Selector2/3 -> Bus Creator2/3  "<acc_z>"
  Bus Creator2/1 -> IMU Data/1

== system PILEncoder/Flight Control Computer/FCC - Real or Emulated/Real FCC/PixBlock2/Emulated Pixhawk/Inertial Navigation System ==
  Enable INS Flag : Inport
  Missile States : Inport  Port=2
  IMU Data : Inport  Port=3
  INS (INCOMPLETE) : Subsystem
  Switch : Switch  Criteria=u2 > Threshold
  INS Data : Outport
  wires:
  Enable INS Flag/1 -> Switch/2
  IMU Data/1 -> INS (INCOMPLETE)/1(IMU Data)
  Switch/1 -> INS Data/1
  Missile States/1 -> Switch/3
  INS (INCOMPLETE)/1(INS Data) -> Switch/1

== system PILEncoder/Flight Control Computer/FCC - Real or Emulated/Real FCC/PixBlock2/Emulated Pixhawk/Real Gyro ==
  HIL Gyro : Inport
  Bus Creator2 : BusCreator  Inputs=3
  Bus Selector2 : BusSelector  OutputSignals=gyro_x,gyro_y,gyro_z
  Gyro Data : Outport
  wires:
  HIL Gyro/1 -> Bus Selector2/1
  Bus Selector2/2 -> Bus Creator2/2  "<gyro_y>"
  Bus Selector2/1 -> Bus Creator2/1  "<gyro_x>"
  Bus Selector2/3 -> Bus Creator2/3  "<gyro_z>"
  Bus Creator2/1 -> Gyro Data/1

== system PILEncoder/Flight Control Computer/FCC - Real or Emulated/Real FCC/PixBlock2/Emulated Pixhawk/Servo Commands ==
  Fin Cmd : Inport
  100Hz Progress : Subsystem
  AND : Logic  IconShape=distinctive  AllPortsSameDT=off  OutDataTypeStr=boolean
  Add{,1..3} (4 alike) : Sum
  Bus Selector : BusSelector  OutputSignals=Fin_1_Cmd_rad,Fin_2_Cmd_rad,Fin_3_Cmd_rad,Fin_4_Cmd_rad
  Cast To Boolean : DataTypeConversion  OutDataTypeStr=boolean
  Cast To Double{,1..3} (4 alike) : DataTypeConversion  OutDataTypeStr=uint16
  Gain{,1..3} (4 alike) : Gain  Gain=1000/91
  One{,1..3} (4 alike) : Constant  Value=1500  OutDataTypeStr=Inherit: Inherit via back propagation
  One4 : Constant  Value=0  OutDataTypeStr=boolean
  PX4 PWM Output1 : px4lib/PX4 PWM Output  pwmDevice=AUX (/dev/pwm_output1)  pwmChannel1_=on  pwmChannel2_=on  pwmChannel3_=on  pwmChannel4_=on  pwmChannel5_=off  pwmChannel6_=off  pwmChannel7_=off  pwmChannel8_=off  forceTerminateFailsafe=off  outputErrorStatus=off
      settings: SourceProductBaseCode=PX4AUTOPILOTS
  Radians to Degrees{,1..3} (4 alike) : simulink_extras/Transformations/Radians to Degrees
  Saturation{,1..3} (4 alike) : Saturate  UpperLimit=20  LowerLimit=-20
  wires:
  Saturation2/1 -> Gain2/1
  Cast To Double3/1 -> PX4 PWM Output1/6
  One4/1 -> PX4 PWM Output1/2
  One/1 -> Add/2
  One2/1 -> Add2/2
  Add1/1 -> Cast To Double1/1
  Gain2/1 -> Add2/1
  AND/1 -> Cast To Boolean/1
  Radians to Degrees1/1 -> Saturation1/1
  Cast To Double2/1 -> PX4 PWM Output1/5
  Add2/1 -> Cast To Double2/1
  Fin Cmd/1 -> Bus Selector/1
  Cast To Double1/1 -> PX4 PWM Output1/4
  Bus Selector/2 -> Radians to Degrees1/1  "<Fin_2_Cmd_rad>"
  Gain/1 -> Add/1
  Bus Selector/4 -> Radians to Degrees3/1  "<Fin_4_Cmd_rad>"
  One3/1 -> Add3/2
  Saturation/1 -> Gain/1
  Gain1/1 -> Add1/1
  Saturation3/1 -> Gain3/1
  Gain3/1 -> Add3/1
  Radians to Degrees3/1 -> Saturation3/1
  Bus Selector/1 -> Radians to Degrees/1  "<Fin_1_Cmd_rad>"
  Bus Selector/3 -> Radians to Degrees2/1  "<Fin_3_Cmd_rad>"
  Saturation1/1 -> Gain1/1
  Cast To Double/1 -> PX4 PWM Output1/3
  Add3/1 -> Cast To Double3/1
  Radians to Degrees2/1 -> Saturation2/1
  [FCC_Enable] -> AND/1
  Radians to Degrees/1 -> Saturation/1
  100Hz Progress/1(RST) -> AND/2
  One1/1 -> Add1/2
  Add/1 -> Cast To Double/1
  Cast To Boolean/1 -> PX4 PWM Output1/1

== system PILEncoder/Non-linear Flight Dynamic Model/Environment/atm_dynamic/trafo_around_z_axis/1_rot_mat/1. Rotation x-Achse ==
  alpha1 : Inport
  Constant : Constant
  Constant{1..2,7..8} (4 alike) : Constant  Value=0
  Gain : Gain  Gain=-1
  Matrix Concatenate : Concatenate  NumInputs=3  Mode=Multidimensional array  ConcatenateDimension=2
  Mux : Mux  Inputs=3
  Mux1 : Mux  Inputs=3
  Mux2 : Mux  Inputs=3
  Trigonometric Function : Trigonometry  Operator=cos
  Trigonometric Function1 : Trigonometry
  Trigonometric Function2 : Trigonometry
  Trigonometric Function3 : Trigonometry  Operator=cos
  1Rot_Matrix_x : Outport  VectorParamsAs1DForOutWhenUnconnected=off
  wires:
  alpha1/1 -> Trigonometric Function2/1, Trigonometric Function/1, Trigonometric Function1/1, Trigonometric Function3/1
  Constant/1 -> Mux/1
  Constant1/1 -> Mux/2
  Constant2/1 -> Mux/3
  Constant8/1 -> Mux1/1
  Trigonometric Function/1 -> Mux1/2
  Trigonometric Function2/1 -> Gain/1
  Constant7/1 -> Mux2/1
  Trigonometric Function1/1 -> Mux2/2
  Trigonometric Function3/1 -> Mux2/3
  Mux/1 -> Matrix Concatenate/1
  Mux1/1 -> Matrix Concatenate/2
  Mux2/1 -> Matrix Concatenate/3
  Matrix Concatenate/1 -> 1Rot_Matrix_x/1
  Gain/1 -> Mux1/3

== system PILEncoder/Non-linear Flight Dynamic Model/Environment/atm_dynamic/trafo_around_z_axis/1_rot_mat/1. Rotation y-Achse ==
  alpha1 : Inport
  Constant{,2,7..8} (4 alike) : Constant  Value=0
  Constant1 : Constant
  Gain1 : Gain  Gain=-1
  Matrix Concatenate : Concatenate  NumInputs=3  Mode=Multidimensional array  ConcatenateDimension=2
  Mux : Mux  Inputs=3
  Mux1 : Mux  Inputs=3
  Mux2 : Mux  Inputs=3
  Trigonometric Function : Trigonometry  Operator=cos
  Trigonometric Function1 : Trigonometry
  Trigonometric Function2 : Trigonometry
  Trigonometric Function3 : Trigonometry  Operator=cos
  1Rot_Matrix_y : Outport  VectorParamsAs1DForOutWhenUnconnected=off
  wires:
  Mux2/1 -> Matrix Concatenate/3
  Mux1/1 -> Matrix Concatenate/2
  Mux/1 -> Matrix Concatenate/1
  Trigonometric Function3/1 -> Mux2/3
  Trigonometric Function1/1 -> Gain1/1
  Constant2/1 -> Mux1/3
  Constant1/1 -> Mux1/2
  Constant/1 -> Mux1/1
  alpha1/1 -> Trigonometric Function1/1, Trigonometric Function3/1, Trigonometric Function2/1, Trigonometric Function/1
  Constant8/1 -> Mux/2
  Trigonometric Function/1 -> Mux/1
  Trigonometric Function2/1 -> Mux/3
  Constant7/1 -> Mux2/2
  Matrix Concatenate/1 -> 1Rot_Matrix_y/1
  Gain1/1 -> Mux2/1

== system PILEncoder/Non-linear Flight Dynamic Model/Environment/atm_dynamic/trafo_around_z_axis/1_rot_mat/1. Rotation z-Achse ==
  alpha1 : Inport
  Constant{4,7..8,10} (4 alike) : Constant  Value=0
  Constant11 : Constant
  Gain : Gain  Gain=-1
  Matrix Concatenate : Concatenate  NumInputs=3  Mode=Multidimensional array  ConcatenateDimension=2
  Mux : Mux  Inputs=3
  Mux1 : Mux  Inputs=3
  Mux2 : Mux  Inputs=3
  Trigonometric Function : Trigonometry  Operator=cos
  Trigonometric Function1 : Trigonometry
  Trigonometric Function3 : Trigonometry  Operator=cos
  Trigonometric Function4 : Trigonometry
  1Rot_Matrix_z : Outport  VectorParamsAs1DForOutWhenUnconnected=off
  wires:
  Trigonometric Function/1 -> Mux1/2
  Mux/1 -> Matrix Concatenate/1
  Mux1/1 -> Matrix Concatenate/2
  Mux2/1 -> Matrix Concatenate/3
  Trigonometric Function1/1 -> Mux1/1
  Constant7/1 -> Mux1/3
  Constant4/1 -> Mux2/1
  Constant10/1 -> Mux2/2
  Constant11/1 -> Mux2/3
  Trigonometric Function3/1 -> Mux/1
  Trigonometric Function4/1 -> Gain/1
  Constant8/1 -> Mux/3
  Matrix Concatenate/1 -> 1Rot_Matrix_z/1
  alpha1/1 -> Trigonometric Function3/1, Trigonometric Function4/1, Trigonometric Function/1, Trigonometric Function1/1
  Gain/1 -> Mux/2

== system PILEncoder/Non-linear Flight Dynamic Model/Extract States/Assemble_States_Bus1/Three-axis Inertial Measurement Unit3/Three-axis Accelerometer/Dynamics ==
  sp_f : Inport
  Constant : Constant  Value=dtype_a
  No Dynamics : Subsystem
  Second-order Dynamics : Subsystem  mask(ContinuousFilter){wn=w_a, zn=z_a}
      mask prompts: wn "Natural frequency:"; zn "Damping ratio:"
      mask init:
      | aeroicon('aeroblk');
  Switch : Switch  Threshold=0.5
  "sp_f " : Outport  VectorParamsAs1DForOutWhenUnconnected=off
  wires:
  Constant/1 -> Switch/2
  Switch/1 -> "sp_f "/1
  Second-order Dynamics/1(Out) -> Switch/1
  No Dynamics/1(Out1) -> Switch/3
  sp_f/1 -> Second-order Dynamics/1(In), No Dynamics/1(In1)
